simulink model "simulationCapstoneLinearMk1"  (R2022b)
settings: Solver=FixedStepAuto  StartTime=0.0  StopTime=10  FixedStep=0.0001  RelTol=1e-3
values from neighbouring files (symbols this model uses):
  A = [0 0 1 0; 0 0 0 1; C1 0 C2 0; 0 C1 0 C2]    [capstoneINIT.m]    (also in controlMathtestScript.m; newPendulumControl.m; timevaryingSYS.m)
  B = [0 0; 0 0; C3 0; 0 C3]    [capstoneINIT.m]    (also in controlMathtestScript.m = eye(4,4); newPendulumControl.m; timevaryingSYS.m)
undefined symbols (not defined in the file or in its folder): K1
settings Model: Creator=rishi  LastModifiedBy=rishi

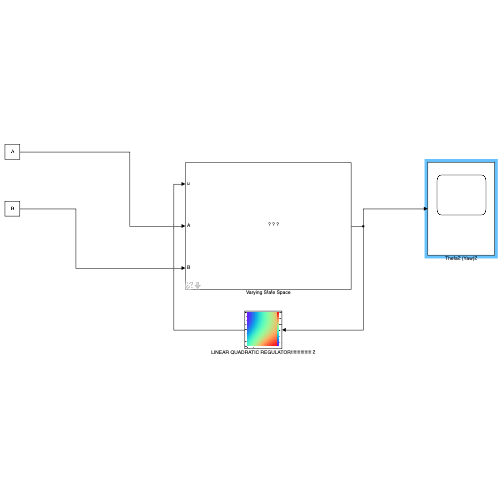
[thumbnail: Simulink's stored preview of the top-level diagram]
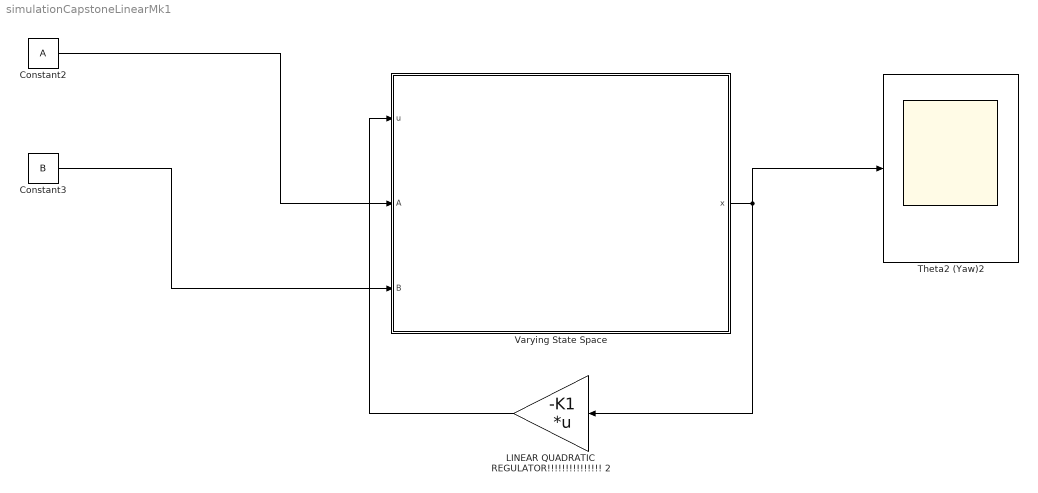
== system simulationCapstoneLinearMk1 ==
  Constant2 : Constant  Value=A  VectorParams1D=off
  Constant3 : Constant  Value=B  VectorParams1D=off
  LINEAR QUADRATIC REGULATOR!!!!!!!!!!!!!!! 2 : Gain  Gain=-K1  Multiplication=Matrix(K*u)
      mask Display: image('/Users/rishi/Desktop/Screen Shot 2022-10-09 at 7.35.45 PM.png'); % Use "Edit Image" on toolstrip to change.
  Theta2 (Yaw)2 : Scope
  Varying State Space : Subsystem  AncestorBlock=cstblocks/Linear Parameter Varying/Varying State Space  mask(Varying State Space){x0=[0.5;0.5;0;0], xNames='', OutputX=on, OutputDX=off}
      mask prompts: x0 "Control:simulink:VaryingSSLabel1"; xNames "Control:simulink:VaryingSSLabel2"; OutputX "Control:simulink:VaryingSSLabel3"; OutputDX "Control:simulink:VaryingSSLabel4"
      mask help: Control:simulink:VaryingSS1
      mask init:
      | % Use exact linearization of product block
      | % pblks = find_system(gcb,'FollowLinks','on',...
      | %    'LookUnderMasks','all','SearchDepth',1,'BlockType','Product');
      | % rep = struct(...
      | %    'Specification','controllib.internal.blocks.matrixProductJacobian',...
      | %    'Type','Function',...
      | %    'ParameterNames','',...
      | %    'ParameterValues','');
      | % for i=1:numel(pblks)
      | %    set_param(pblks{i},...
      | %       'SCDEnableBlockLinearizationSpecification','on',...
      | %       'SCDBlockLinearizationSpecification',rep)
      | % end
      | SimStatus = get_param(bdroot,'SimulationStatus');
      | if any(strcmp(SimStatus,{'initializing','updating','stopped'}))
      |    varyingBlockMask('ss',gcb,OutputX,OutputDX)
      | end
      settings: LibrarySourceBlock=cstblocks/Linear Parameter Varying/Varying State Space
      mask Help: eval('ctrlguihelp(''VaryingSSCT'');')
      mask DialogControl x0 Prompt: Initial conditions:
      mask DialogControl xNames Prompt: State names (e.g., 'position'):
      mask DialogControl OutputX Prompt: Output states
      mask DialogControl OutputDX Prompt: Output state derivatives
      mask Display:
      | port_label('input', 1, 'u')
      | port_label('input', 2, 'A')
      | port_label('input', 3, 'B')
      | port_label('input', 4, 'C')
      | port_label('input', 5, 'D')
      | port_label('output', 1, 'y')
      | next_ = 2;
      | if OutputX
      |    port_label('output', next_, 'x')
      |    next_ = next_+1;
      | end
      | if OutputDX
      |    port_label('output', next_, 'dx')
      |    next_ = next_+1;
      | end
      | text(0.5,0.65,'dx = A x + B u',...
      |    'horizontalAlignment', 'center','texmode','on')
      | text(0.5,0.35,'y = C x + D u',...
      |    'horizontalAlignment', 'center','texmode','on')
  wires:
  Constant2/1 -> Varying State Space/2(A)
  Constant3/1 -> Varying State Space/3(B)
  LINEAR QUADRATIC REGULATOR!!!!!!!!!!!!!!! 2/1 -> Varying State Space/1(u)
  Varying State Space/1(x) -> Theta2 (Yaw)2/1, LINEAR QUADRATIC REGULATOR!!!!!!!!!!!!!!! 2/1

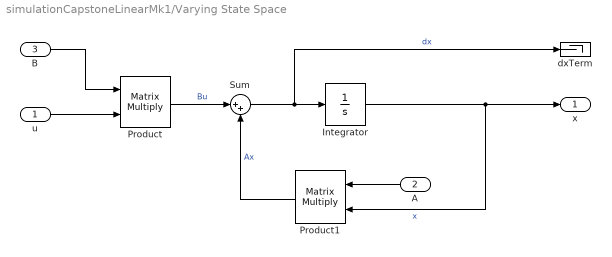
== system simulationCapstoneLinearMk1/Varying State Space ==
  u : Inport
  A : Inport  Port=2
  B : Inport  Port=3
  Integrator : Integrator  InitialCondition=x0  ContinuousStateAttributes=xNames
  Product : Product  SCDEnableBlockLinearizationSpecification=on  Multiplication=Matrix(*)
  Product1 : Product  SCDEnableBlockLinearizationSpecification=on  Multiplication=Matrix(*)
  Sum : Sum  Inputs=|++
  dxTerm : Terminator
  x : Outport
  wires:
  u/1 -> Product/2
  A/1 -> Product1/1
  Product1/1 -> Sum/2  "Ax"
  B/1 -> Product/1
  Integrator/1 -> x/1, Product1/2  "x"
  Sum/1 -> Integrator/1, dxTerm/1  "dx"
  Product/1 -> Sum/1  "Bu"
